simulink model "simulinkDroneDynamics"  (R2022b)
settings: Solver=VariableStepAuto  StartTime=0.0  StopTime=10.0  FixedStep=dt  RelTol=1e-3
values from neighbouring files (symbols this model uses):
  b = 0.71    [Data.m]
  g_vect = [0; 0; m*g]    [Data.m]
  Kd_vx = 0.5    [Data.m]
  Kd_vy = 0.5    [Data.m]
  Kd_vz = 1    [Data.m]
  Ki_vx = 0.5    [Data.m]
  Ki_vy = 0.5    [Data.m]
  Ki_vz = 10    [Data.m]
  Kp_vx = 5    [Data.m]
  Kp_vy = 5    [Data.m]
  Kp_vz = 15    [Data.m]
  Kp_x = 0.1    [Data.m]
  Kp_y = 0.1    [Data.m]
  Kp_z = 1    [Data.m]
  m = 3.074    [Data.m]
  mixer = [        -1         -1        -1         -1 ... (first row only)    [Data.m]
  mixer_inv = inv(mixer)    [Data.m]
  NED2ECI = [ 1  0  0 ... (first row only)    [Data.m]
  omega0 = zeros(3,1)    [Data.m]
  p0 = zeros(3,1)    [Data.m]
  q0 = [1 0 0 0]'    [Data.m]
  tau = 1/900    (= 0.00111111111111)    [Data.m]
  v0 = zeros(3,1)    [Data.m]
undefined symbols (not defined in the file or in its folder): guidance
libraries: slpidlib x3, sharedtransform x1, simulink_extras x1, sim3dlib x1, uavsim3dlib x1
settings Model: Creator=Pietro Bruschi  LastModifiedBy=Utente
settings SFSimCC: SimCustomHeaderCode="#include \"controller_vel.h\""  SimUserSources=controller_vel.c  CustomCodeGlobalsAsFunctionIO=on

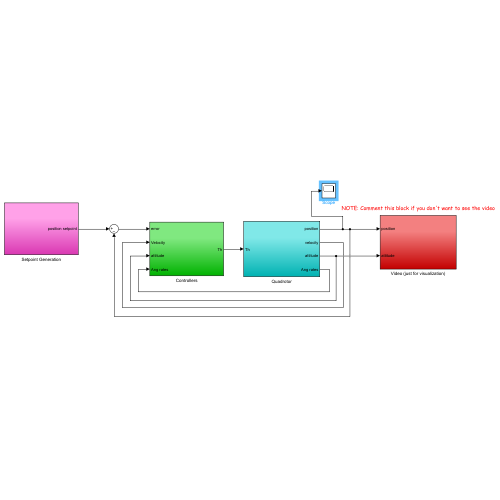
[thumbnail: Simulink's stored preview of the top-level diagram]
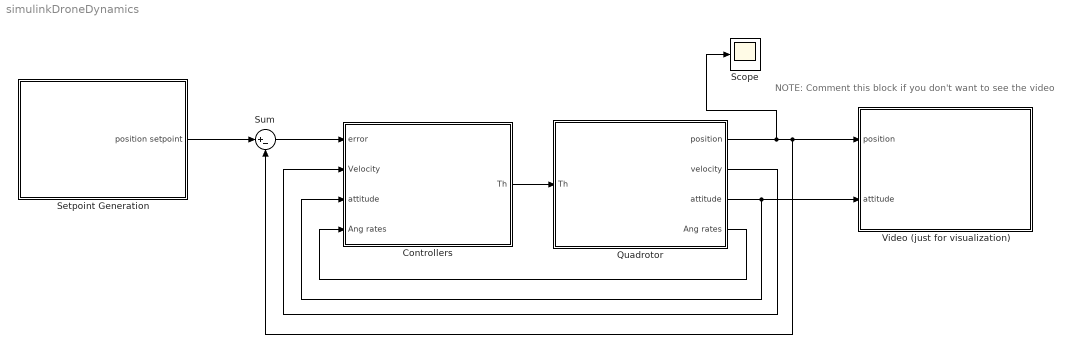
== system simulinkDroneDynamics ==
  note: NOTE: Comment this block if you don't want to see the video
  Controllers : Subsystem
  Quadrotor : Subsystem
  Scope : Scope
  Setpoint Generation : Subsystem
  Sum : Sum  Inputs=|+-
  Video (just for visualization) : Subsystem
  wires:
  Sum/1 -> Controllers/1("error ")
  Controllers/1(Th) -> Quadrotor/1(Th)
  Quadrotor/1(position) -> Scope/1, Sum/2, Video (just for visualization)/1(position)
  Setpoint Generation/1(position setpoint) -> Sum/1
  Quadrotor/4(Ang rates) -> Controllers/4(Ang rates)
  Quadrotor/3(attitude) -> Controllers/3(attitude), Video (just for visualization)/2(attitude)
  Quadrotor/2(velocity) -> Controllers/2(Velocity)

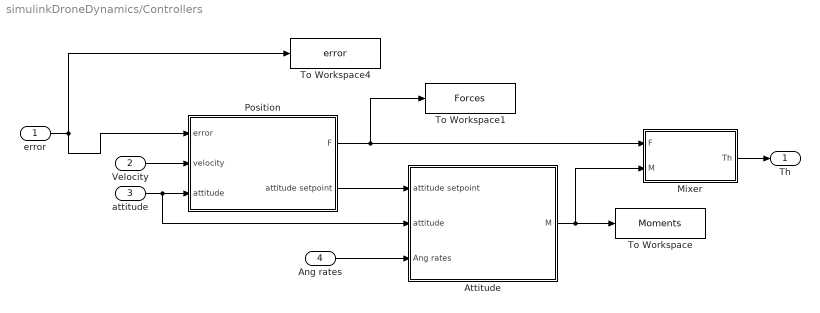
== system simulinkDroneDynamics/Controllers ==
  "error " : Inport
  Velocity : Inport  Port=2
  attitude : Inport  Port=3
  Ang rates : Inport  Port=4
  Attitude : Subsystem
  Mixer : Subsystem
  Position : Subsystem
  To Workspace : ToWorkspace  VariableName=Moments  SaveFormat=Timeseries  SampleTime=-1
  To Workspace1 : ToWorkspace  VariableName=Forces  SaveFormat=Timeseries  SampleTime=-1
  To Workspace4 : ToWorkspace  VariableName=error  SaveFormat=Timeseries  SampleTime=-1
  Th : Outport
  wires:
  Position/2(attitude setpoint) -> Attitude/1(attitude setpoint)
  Velocity/1 -> Position/2(velocity)
  Attitude/1(M) -> Mixer/2(M), To Workspace/1
  attitude/1 -> Position/3(attitude), Attitude/2(attitude)
  Ang rates/1 -> Attitude/3(Ang rates)
  Position/1(F) -> Mixer/1(F), To Workspace1/1
  Mixer/1(Th) -> Th/1
  "error "/1 -> Position/1("error "), To Workspace4/1

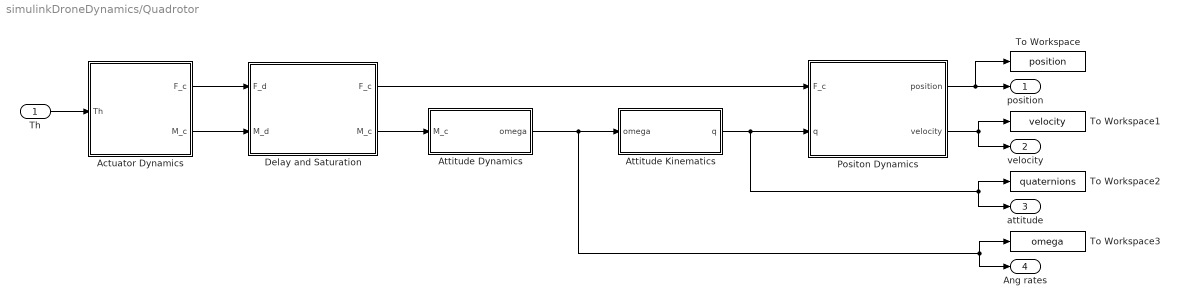
== system simulinkDroneDynamics/Quadrotor ==
  Th : Inport
  Actuator Dynamics : Subsystem
  Attitude Dynamics : Subsystem
  Attitude Kinematics : Subsystem
  Delay and Saturation : Subsystem
  Positon Dynamics : Subsystem
  To Workspace : ToWorkspace  VariableName=position  SaveFormat=Timeseries  SampleTime=-1
  To Workspace1 : ToWorkspace  VariableName=velocity  SaveFormat=Timeseries  SampleTime=-1
  To Workspace2 : ToWorkspace  VariableName=quaternions  SaveFormat=Timeseries  SampleTime=-1
  To Workspace3 : ToWorkspace  VariableName=omega  SaveFormat=Timeseries  SampleTime=-1
  position : Outport
  velocity : Outport  Port=2
  attitude : Outport  Port=3
  Ang rates : Outport  Port=4
  wires:
  Attitude Dynamics/1(omega) -> To Workspace3/1, Ang rates/1, Attitude Kinematics/1(omega)
  Attitude Kinematics/1(q) -> To Workspace2/1, attitude/1, Positon Dynamics/2(q)
  Positon Dynamics/1(position) -> To Workspace/1, position/1
  Positon Dynamics/2(velocity) -> velocity/1, To Workspace1/1
  Th/1 -> Actuator Dynamics/1(Th)
  Delay and Saturation/2(M_c) -> Attitude Dynamics/1(M_c)
  Actuator Dynamics/2(M_c) -> Delay and Saturation/2(M_d)
  Actuator Dynamics/1(F_c) -> Delay and Saturation/1(F_d)
  Delay and Saturation/1(F_c) -> Positon Dynamics/1(F_c)

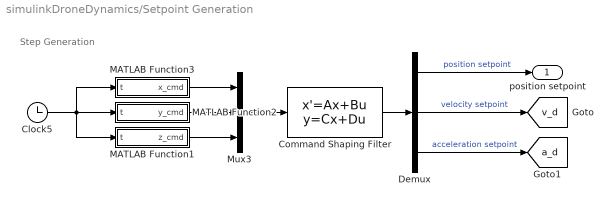
== system simulinkDroneDynamics/Setpoint Generation ==
  note: Step Generation
  Clock5 : Clock
  "Command Shaping Filter " : StateSpace  A=guidance.A_d  B=guidance.B_d  C=eye(9)  D=zeros(9,3)  InitialCondition=zeros(9,1)
  Demux : Demux  Outputs=3
  MATLAB Function1 : MATLAB Function  TreatAsAtomicUnit=on
  MATLAB Function2 : MATLAB Function  TreatAsAtomicUnit=on
  MATLAB Function3 : MATLAB Function  TreatAsAtomicUnit=on
  Mux3 : Mux  Inputs=3
  position setpoint : Outport
  tag scope: a_d=global, v_d=global
  wires:
  MATLAB Function1/1(z_cmd) -> Mux3/3
  MATLAB Function3/1(x_cmd) -> Mux3/1
  "Command Shaping Filter "/1 -> Demux/1
  Mux3/1 -> "Command Shaping Filter "/1
  MATLAB Function2/1(y_cmd) -> Mux3/2
  Clock5/1 -> MATLAB Function1/1(t), MATLAB Function2/1(t), MATLAB Function3/1(t)
  Demux/2 -> [v_d]  "velocity setpoint"
  Demux/3 -> [a_d]  "acceleration setpoint"
  Demux/1 -> position setpoint/1  "position setpoint"

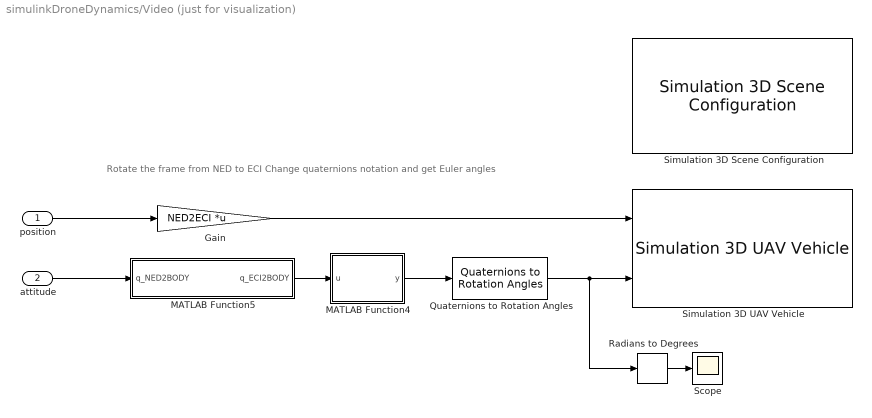
== system simulinkDroneDynamics/Video (just for visualization) ==
  note: Rotate the frame from NED to ECI
      | Change quaternions notation and get Euler angles
  position : Inport
  attitude : Inport  Port=2
  Gain : Gain  Gain=NED2ECI  Multiplication=Matrix(K*u)
  MATLAB Function4 : MATLAB Function  TreatAsAtomicUnit=on
  MATLAB Function5 : MATLAB Function  TreatAsAtomicUnit=on
  Quaternions to Rotation Angles : sharedtransform/Quaternions to Rotation Angles  rotationOrder=ZYX  aMode=aMode
  Radians to Degrees : simulink_extras/Transformations/Radians to Degrees
  Scope : Scope
  Simulation 3D Scene Configuration : sim3dlib/Simulation 3D Scene Configuration  Priority=0  ProjectFormat=Default Scenes  SceneDesc=US city block  ProjectName=C:\Program Files\MATLAB\R2022b\toolbox\shared\sim3d_projects\automotive_project\UE4\WindowsNoEditor\VehicleSimulation.exe  ScenePath=/Game/Maps/USCityBlock  EnableOpenDRIVE=off  vehTagList={'Scene Origin';'SimulinkVehicle1'}  vehTag=Scene Origin  OpVisEn=off  Ts=0.01  EnableWindow=on  EnableRemoteAccess=off  EnableWeather=off  SunAltitude=40.0  SunAzimuth=90  clouds=10  wind=1  fog=0  rain=0  EnableGeospatial=off  OriginHeight=200  OriginLatitude=40.744652  OriginLongitude=-73.988864  MapStyle=Aerial  AdditionalAssetIDs=[]  UseAdvancedSunSky=off  SolarTime=11  TimeZone=-5  Day=21  Month=9  Year=2022  UseDaylightSavingTime=on  DSTStartDay=10  DSTStartMonth=3  DSTEndDay=3  DSTEndMonth=11  DSTSwitchHour=2  sensorTag=MainCamera1  sensorId=1  sensorName=MainCamera1  mountLoc=Origin  offsetFlag=off  tmountOffset=[0, 0, 0]  rmountOffset=[0, 0, 0]  HorizontalResolution=1280  VerticalResolution=720  HorizontalFOV=60  mountPoint=[0 0 0]  mountOrientation=[0 0 0]  aMode=4  ID=1  GeoTrigger=Inactive
      settings: LibrarySourceBlock=uavsim3dlib/Simulation 3D Scene Configuration
  Simulation 3D UAV Vehicle : uavsim3dlib/Simulation 3D UAV Vehicle  Priority=-1  Mesh=Quadrotor  MeshPath=/MathWorksUAVContent/UAVs/HexaRotorUAV/HexaRotor.HexaRotor  Color=Black  ActorName=SimulinkVehicle1  InitialTranslation=[0 0 .2]  InitialRotation=[0 0 0]  SampleTime=-1  ActorType=SimulinkVehicle  ID=1  aMode=4  ActorTag=SimulinkVehicle1
  wires:
  Radians to Degrees/1 -> Scope/1
  MATLAB Function5/1(q_ECI2BODY) -> MATLAB Function4/1(u)
  position/1 -> Gain/1
  MATLAB Function4/1(y) -> Quaternions to Rotation Angles/1
  Gain/1 -> Simulation 3D UAV Vehicle/1
  attitude/1 -> MATLAB Function5/1(q_NED2BODY)
  Quaternions to Rotation Angles/1 -> Simulation 3D UAV Vehicle/2, Radians to Degrees/1

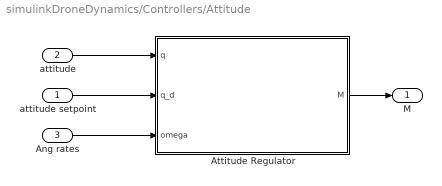
== system simulinkDroneDynamics/Controllers/Attitude ==
  attitude setpoint : Inport
  attitude : Inport  Port=2
  Ang rates : Inport  Port=3
  Attitude Regulator : MATLAB Function  TreatAsAtomicUnit=on
  M : Outport
  wires:
  attitude/1 -> Attitude Regulator/1(q)
  Attitude Regulator/1(M) -> M/1
  Ang rates/1 -> Attitude Regulator/3(omega)
  attitude setpoint/1 -> Attitude Regulator/2(q_d)

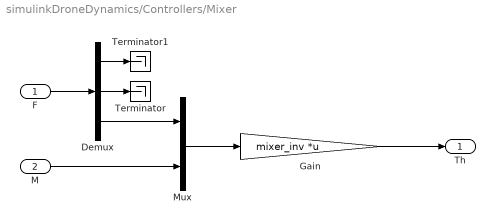
== system simulinkDroneDynamics/Controllers/Mixer ==
  F : Inport
  M : Inport  Port=2
  Demux : Demux  Outputs=3
  Gain : Gain  Gain=mixer_inv  Multiplication=Matrix(K*u) (u vector)
  Mux : Mux  Inputs=2
  Terminator : Terminator
  Terminator1 : Terminator
  Th : Outport
  wires:
  M/1 -> Mux/2
  Mux/1 -> Gain/1
  Demux/3 -> Mux/1
  F/1 -> Demux/1
  Demux/2 -> Terminator/1
  Demux/1 -> Terminator1/1
  Gain/1 -> Th/1

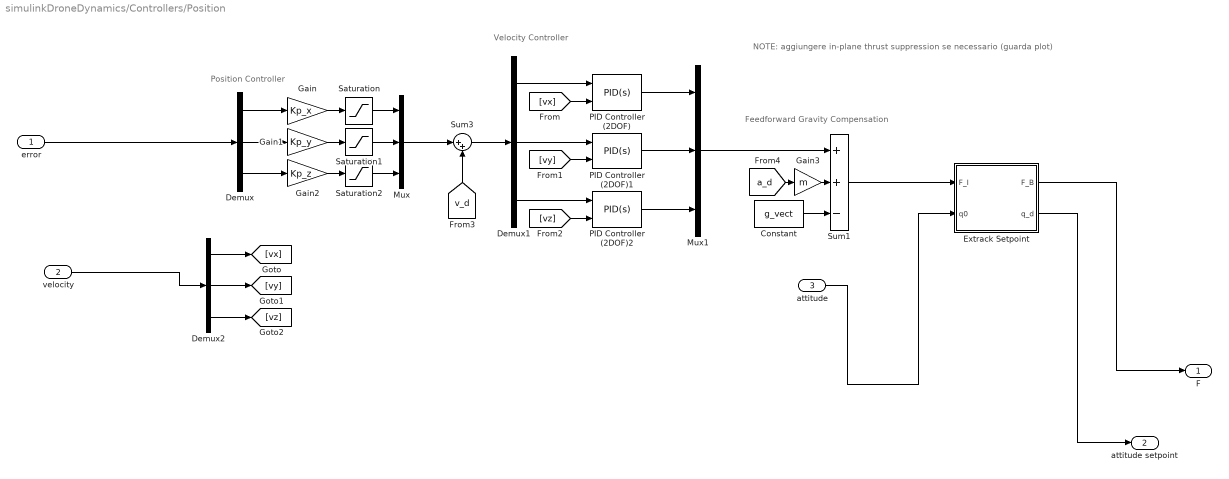
== system simulinkDroneDynamics/Controllers/Position ==
  note: Feedforward Gravity
      | Compensation
  note: NOTE: aggiungere in-plane thrust suppression se necessario (guarda plot)
  note: Velocity Controller
  note: Position Controller
  "error " : Inport
  velocity : Inport  Port=2
  attitude : Inport  Port=3
  Constant : Constant  Value=g_vect
  Demux : Demux  Outputs=3
  Demux1 : Demux  Outputs=3
  Demux2 : Demux  Outputs=3
  Extrack Setpoint : MATLAB Function  TreatAsAtomicUnit=on
  Gain : Gain  Gain=Kp_x
  Gain1 : Gain  Gain=Kp_y
  Gain2 : Gain  Gain=Kp_z
  Gain3 : Gain  Gain=m
  Mux : Mux  Inputs=3
  Mux1 : Mux  Inputs=3
  PID Controller (2DOF) : slpidlib/PID Controller (2DOF)  Controller=PID  Form=Parallel  TimeDomain=Continuous-time  UseExternalTs=off  SampleTime=-1  IntegratorMethod=Forward Euler  FilterMethod=Forward Euler  ControllerParametersSource=internal  P=Kp_vx  I=Ki_vx  UseKiTs=off  D=Kd_vx  N=100  UseFilter=on  b=1  c=0  TunerSelectOption=Frequency Response Based  InitialConditionSource=internal  InitialConditionForIntegrator=0  InitialConditionForFilter=0  DifferentiatorICPrevScaledInput=0  ExternalReset=none  TrackingMode=off  Kt=1  LimitOutput=off  SatLimitsSource=internal  UpperSaturationLimit=inf  LowerSaturationLimit=-inf  LinearizeAsGain=on  AntiWindupMode=none  Kb=1  LimitIntegrator=off  UpperIntegratorSaturationLimit=inf  LowerIntegratorSaturationLimit=-inf  POutMin=[]  POutMax=[]  IOutMin=[]  IOutMax=[]  DOutMin=[]  DOutMax=[]  NOutMin=[]  NOutMax=[]  bOutMin=[]  bOutMax=[]  cOutMin=[]  cOutMax=[]  SumOutMin=[]  SumOutMax=[]  SaturationOutMin=[]  SaturationOutMax=[]  PParamMin=[]  PParamMax=[]  IParamMin=[]  IParamMax=[]  DParamMin=[]  DParamMax=[]  NParamMin=[]  NParamMax=[]  bParamMin=[]  bParamMax=[]  cParamMin=[]  cParamMax=[]  KbParamMin=[]  KbParamMax=[]  KtParamMin=[]  KtParamMax=[]  KbOutMin=[]  KbOutMax=[]  KtOutMin=[]  KtOutMax=[]  IntegratorOutMin=[]  IntegratorOutMax=[]  FilterOutMin=[]  FilterOutMax=[]  SumI1OutMin=[]  SumI1OutMax=[]  SumI2OutMin=[]  SumI2OutMax=[]  SumI3OutMin=[]  SumI3OutMax=[]  SumI4OutMin=[]  SumI4OutMax=[]  SumDOutMin=[]  SumDOutMax=[]  Sum1OutMin=[]  Sum1OutMax=[]  Sum2OutMin=[]  Sum2OutMax=[]  Sum3OutMin=[]  Sum3OutMax=[]  DifferentiatorOutMin=[]  DifferentiatorOutMax=[]  FilterDiffOutCoefMin=[]  FilterDiffOutCoefMax=[]  ReciprocalOutMin=[]  ReciprocalOutMax=[]  SumDenOutMin=[]  SumDenOutMax=[]  SumNumOutMin=[]  SumNumOutMax=[]  DivideOutMin=[]  DivideOutMax=[]  UdiffTsProdOutMin=[]  UdiffTsProdOutMax=[]  NTsProdOutMin=[]  NTsProdOutMax=[]  UintegralTsProdOutMin=[]  UintegralTsProdOutMax=[]  UngainTsProdOutMin=[]  UngainTsProdOutMax=[]  ClampingZeroOutDataTypeStr=Inherit: Inherit via back propagation  ClampingZeroOutMin=[]  ClampingZeroOutMax=[]  FilterDenConstantOutDataTypeStr=Inherit: Inherit via back propagation  FilterDenConstantOutMin=[]  FilterDenConstantOutMax=[]  PCopyOutDataTypeStr=Inherit: Inherit via back propagation  PCopyOutMin=[]  PCopyOutMax=[]  NCopyOutDataTypeStr=Inherit: Inherit via back propagation  NCopyOutMin=[]  NCopyOutMax=[]  IntegratorContinuousStateAttributes=''  IntegratorStateMustResolveToSignalObject=off  IntegratorRTWStateStorageClass=Auto  FilterContinuousStateAttributes=''  FilterStateMustResolveToSignalObject=off  FilterRTWStateStorageClass=Auto  ParallelPVariant=InternalParameters  IdealPVariant=Disabled  IVariant=InternalParameters  DVariant=InternalParameters  bVariant=InternalParameters  cVariant=InternalParameters  IntegratorVariant=Continuous  SatVariant=Disabled  AWVariant=Passthrough  PCopyVariant=Disabled  TRVariant=Disabled  FdbkBlocksVariant=Forward  IdealPFdbkVariant=Disabled  SatFdbkVariant=Disabled  DerivativeFilterVariant=ContFilter  NVariant=InternalParameters  NCopyVariant=Disabled  FilterICVariant=InternalICsFilter  IntegratorICVariant=InternalICs  ExternalResetVariant=Disabled  TRSumVariant=Passthrough  SumFdbkVariant=Disabled  SumVariant=Sum_PID  TsampFilterVariant=InternalTs  TsampNgainVariant=Passthrough  TsampIntegralVariant=Passthrough  ExternalSaturationOutDataTypeStr=Inherit: Same as second input
  PID Controller (2DOF)1 : slpidlib/PID Controller (2DOF)  Controller=PID  Form=Parallel  TimeDomain=Continuous-time  UseExternalTs=off  SampleTime=-1  IntegratorMethod=Forward Euler  FilterMethod=Forward Euler  ControllerParametersSource=internal  P=Kp_vy  I=Ki_vy  UseKiTs=off  D=Kd_vy  N=100  UseFilter=on  b=1  c=0  TunerSelectOption=Frequency Response Based  InitialConditionSource=internal  InitialConditionForIntegrator=0  InitialConditionForFilter=0  DifferentiatorICPrevScaledInput=0  ExternalReset=none  TrackingMode=off  Kt=1  LimitOutput=off  SatLimitsSource=internal  UpperSaturationLimit=inf  LowerSaturationLimit=-inf  LinearizeAsGain=on  AntiWindupMode=none  Kb=1  LimitIntegrator=off  UpperIntegratorSaturationLimit=inf  LowerIntegratorSaturationLimit=-inf  POutMin=[]  POutMax=[]  IOutMin=[]  IOutMax=[]  DOutMin=[]  DOutMax=[]  NOutMin=[]  NOutMax=[]  bOutMin=[]  bOutMax=[]  cOutMin=[]  cOutMax=[]  SumOutMin=[]  SumOutMax=[]  SaturationOutMin=[]  SaturationOutMax=[]  PParamMin=[]  PParamMax=[]  IParamMin=[]  IParamMax=[]  DParamMin=[]  DParamMax=[]  NParamMin=[]  NParamMax=[]  bParamMin=[]  bParamMax=[]  cParamMin=[]  cParamMax=[]  KbParamMin=[]  KbParamMax=[]  KtParamMin=[]  KtParamMax=[]  KbOutMin=[]  KbOutMax=[]  KtOutMin=[]  KtOutMax=[]  IntegratorOutMin=[]  IntegratorOutMax=[]  FilterOutMin=[]  FilterOutMax=[]  SumI1OutMin=[]  SumI1OutMax=[]  SumI2OutMin=[]  SumI2OutMax=[]  SumI3OutMin=[]  SumI3OutMax=[]  SumI4OutMin=[]  SumI4OutMax=[]  SumDOutMin=[]  SumDOutMax=[]  Sum1OutMin=[]  Sum1OutMax=[]  Sum2OutMin=[]  Sum2OutMax=[]  Sum3OutMin=[]  Sum3OutMax=[]  DifferentiatorOutMin=[]  DifferentiatorOutMax=[]  FilterDiffOutCoefMin=[]  FilterDiffOutCoefMax=[]  ReciprocalOutMin=[]  ReciprocalOutMax=[]  SumDenOutMin=[]  SumDenOutMax=[]  SumNumOutMin=[]  SumNumOutMax=[]  DivideOutMin=[]  DivideOutMax=[]  UdiffTsProdOutMin=[]  UdiffTsProdOutMax=[]  NTsProdOutMin=[]  NTsProdOutMax=[]  UintegralTsProdOutMin=[]  UintegralTsProdOutMax=[]  UngainTsProdOutMin=[]  UngainTsProdOutMax=[]  ClampingZeroOutDataTypeStr=Inherit: Inherit via back propagation  ClampingZeroOutMin=[]  ClampingZeroOutMax=[]  FilterDenConstantOutDataTypeStr=Inherit: Inherit via back propagation  FilterDenConstantOutMin=[]  FilterDenConstantOutMax=[]  PCopyOutDataTypeStr=Inherit: Inherit via back propagation  PCopyOutMin=[]  PCopyOutMax=[]  NCopyOutDataTypeStr=Inherit: Inherit via back propagation  NCopyOutMin=[]  NCopyOutMax=[]  IntegratorContinuousStateAttributes=''  IntegratorStateMustResolveToSignalObject=off  IntegratorRTWStateStorageClass=Auto  FilterContinuousStateAttributes=''  FilterStateMustResolveToSignalObject=off  FilterRTWStateStorageClass=Auto  ParallelPVariant=InternalParameters  IdealPVariant=Disabled  IVariant=InternalParameters  DVariant=InternalParameters  bVariant=InternalParameters  cVariant=InternalParameters  IntegratorVariant=Continuous  SatVariant=Disabled  AWVariant=Passthrough  PCopyVariant=Disabled  TRVariant=Disabled  FdbkBlocksVariant=Forward  IdealPFdbkVariant=Disabled  SatFdbkVariant=Disabled  DerivativeFilterVariant=ContFilter  NVariant=InternalParameters  NCopyVariant=Disabled  FilterICVariant=InternalICsFilter  IntegratorICVariant=InternalICs  ExternalResetVariant=Disabled  TRSumVariant=Passthrough  SumFdbkVariant=Disabled  SumVariant=Sum_PID  TsampFilterVariant=InternalTs  TsampNgainVariant=Passthrough  TsampIntegralVariant=Passthrough  ExternalSaturationOutDataTypeStr=Inherit: Same as second input
  PID Controller (2DOF)2 : slpidlib/PID Controller (2DOF)  Controller=PID  Form=Parallel  TimeDomain=Continuous-time  UseExternalTs=off  SampleTime=-1  IntegratorMethod=Forward Euler  FilterMethod=Forward Euler  ControllerParametersSource=internal  P=Kp_vz  I=Ki_vz  UseKiTs=off  D=Kd_vz  N=100  UseFilter=on  b=1  c=0  TunerSelectOption=Frequency Response Based  InitialConditionSource=internal  InitialConditionForIntegrator=0  InitialConditionForFilter=0  DifferentiatorICPrevScaledInput=0  ExternalReset=none  TrackingMode=off  Kt=1  LimitOutput=off  SatLimitsSource=internal  UpperSaturationLimit=inf  LowerSaturationLimit=-inf  LinearizeAsGain=on  AntiWindupMode=none  Kb=1  LimitIntegrator=off  UpperIntegratorSaturationLimit=inf  LowerIntegratorSaturationLimit=-inf  POutMin=[]  POutMax=[]  IOutMin=[]  IOutMax=[]  DOutMin=[]  DOutMax=[]  NOutMin=[]  NOutMax=[]  bOutMin=[]  bOutMax=[]  cOutMin=[]  cOutMax=[]  SumOutMin=[]  SumOutMax=[]  SaturationOutMin=[]  SaturationOutMax=[]  PParamMin=[]  PParamMax=[]  IParamMin=[]  IParamMax=[]  DParamMin=[]  DParamMax=[]  NParamMin=[]  NParamMax=[]  bParamMin=[]  bParamMax=[]  cParamMin=[]  cParamMax=[]  KbParamMin=[]  KbParamMax=[]  KtParamMin=[]  KtParamMax=[]  KbOutMin=[]  KbOutMax=[]  KtOutMin=[]  KtOutMax=[]  IntegratorOutMin=[]  IntegratorOutMax=[]  FilterOutMin=[]  FilterOutMax=[]  SumI1OutMin=[]  SumI1OutMax=[]  SumI2OutMin=[]  SumI2OutMax=[]  SumI3OutMin=[]  SumI3OutMax=[]  SumI4OutMin=[]  SumI4OutMax=[]  SumDOutMin=[]  SumDOutMax=[]  Sum1OutMin=[]  Sum1OutMax=[]  Sum2OutMin=[]  Sum2OutMax=[]  Sum3OutMin=[]  Sum3OutMax=[]  DifferentiatorOutMin=[]  DifferentiatorOutMax=[]  FilterDiffOutCoefMin=[]  FilterDiffOutCoefMax=[]  ReciprocalOutMin=[]  ReciprocalOutMax=[]  SumDenOutMin=[]  SumDenOutMax=[]  SumNumOutMin=[]  SumNumOutMax=[]  DivideOutMin=[]  DivideOutMax=[]  UdiffTsProdOutMin=[]  UdiffTsProdOutMax=[]  NTsProdOutMin=[]  NTsProdOutMax=[]  UintegralTsProdOutMin=[]  UintegralTsProdOutMax=[]  UngainTsProdOutMin=[]  UngainTsProdOutMax=[]  ClampingZeroOutDataTypeStr=Inherit: Inherit via back propagation  ClampingZeroOutMin=[]  ClampingZeroOutMax=[]  FilterDenConstantOutDataTypeStr=Inherit: Inherit via back propagation  FilterDenConstantOutMin=[]  FilterDenConstantOutMax=[]  PCopyOutDataTypeStr=Inherit: Inherit via back propagation  PCopyOutMin=[]  PCopyOutMax=[]  NCopyOutDataTypeStr=Inherit: Inherit via back propagation  NCopyOutMin=[]  NCopyOutMax=[]  IntegratorContinuousStateAttributes=''  IntegratorStateMustResolveToSignalObject=off  IntegratorRTWStateStorageClass=Auto  FilterContinuousStateAttributes=''  FilterStateMustResolveToSignalObject=off  FilterRTWStateStorageClass=Auto  ParallelPVariant=InternalParameters  IdealPVariant=Disabled  IVariant=InternalParameters  DVariant=InternalParameters  bVariant=InternalParameters  cVariant=InternalParameters  IntegratorVariant=Continuous  SatVariant=Disabled  AWVariant=Passthrough  PCopyVariant=Disabled  TRVariant=Disabled  FdbkBlocksVariant=Forward  IdealPFdbkVariant=Disabled  SatFdbkVariant=Disabled  DerivativeFilterVariant=ContFilter  NVariant=InternalParameters  NCopyVariant=Disabled  FilterICVariant=InternalICsFilter  IntegratorICVariant=InternalICs  ExternalResetVariant=Disabled  TRSumVariant=Passthrough  SumFdbkVariant=Disabled  SumVariant=Sum_PID  TsampFilterVariant=InternalTs  TsampNgainVariant=Passthrough  TsampIntegralVariant=Passthrough  ExternalSaturationOutDataTypeStr=Inherit: Same as second input
  Saturation : Saturate  UpperLimit=10  LowerLimit=-10
  Saturation1 : Saturate  UpperLimit=10  LowerLimit=-10
  Saturation2 : Saturate  UpperLimit=10  LowerLimit=-10
  Sum1 : Sum  Inputs=++-
  Sum3 : Sum  Inputs=|++
  F : Outport
  attitude setpoint : Outport  Port=2
  wires:
  Demux/1 -> Gain/1
  Demux/2 -> Gain1/1
  Demux/3 -> Gain2/1
  Demux2/1 -> [vx]
  Demux2/2 -> [vy]
  Demux2/3 -> [vz]
  "error "/1 -> Demux/1
  velocity/1 -> Demux2/1
  attitude/1 -> Extrack Setpoint/2(q0)
  Gain1/1 -> Saturation1/1
  Gain2/1 -> Saturation2/1
  Gain/1 -> Saturation/1
  Sum1/1 -> Extrack Setpoint/1(F_I)
  PID Controller (2DOF)1/1 -> Mux1/2
  Demux1/2 -> PID Controller (2DOF)1/1
  [vy] -> PID Controller (2DOF)1/2
  Saturation1/1 -> Mux/2
  Saturation2/1 -> Mux/3
  Saturation/1 -> Mux/1
  Mux/1 -> Sum3/1
  Sum3/1 -> Demux1/1
  [v_d] -> Sum3/2
  Constant/1 -> Sum1/3
  Gain3/1 -> Sum1/2
  [a_d] -> Gain3/1
  PID Controller (2DOF)2/1 -> Mux1/3
  Demux1/3 -> PID Controller (2DOF)2/1
  [vz] -> PID Controller (2DOF)2/2
  Mux1/1 -> Sum1/1
  PID Controller (2DOF)/1 -> Mux1/1
  Demux1/1 -> PID Controller (2DOF)/1
  [vx] -> PID Controller (2DOF)/2
  Extrack Setpoint/1(F_B) -> F/1
  Extrack Setpoint/2(q_d) -> attitude setpoint/1

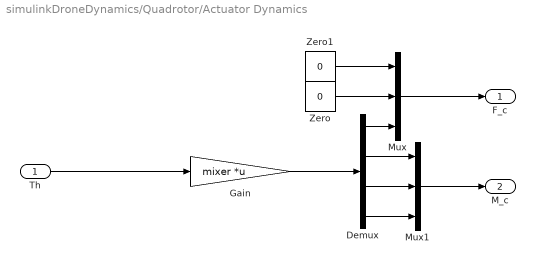
== system simulinkDroneDynamics/Quadrotor/Actuator Dynamics ==
  Th : Inport
  Demux : Demux
  Gain : Gain  Gain=mixer  Multiplication=Matrix(K*u) (u vector)
  Mux : Mux  Inputs=3
  Mux1 : Mux  Inputs=3
  Zero : Constant  Value=0  OutDataTypeStr=Inherit: Inherit via back propagation
  Zero1 : Constant  Value=0  OutDataTypeStr=Inherit: Inherit via back propagation
  F_c : Outport
  M_c : Outport  Port=2
  wires:
  Gain/1 -> Demux/1
  Mux/1 -> F_c/1
  Demux/1 -> Mux/3
  Zero1/1 -> Mux/1
  Zero/1 -> Mux/2
  Mux1/1 -> M_c/1
  Demux/2 -> Mux1/1
  Demux/3 -> Mux1/2
  Demux/4 -> Mux1/3
  Th/1 -> Gain/1

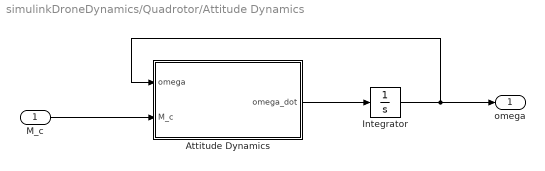
== system simulinkDroneDynamics/Quadrotor/Attitude Dynamics ==
  M_c : Inport
  Attitude Dynamics : MATLAB Function  TreatAsAtomicUnit=on
  Integrator : Integrator  InitialCondition=omega0
  omega : Outport
  wires:
  M_c/1 -> Attitude Dynamics/2(M_c)
  Attitude Dynamics/1(omega_dot) -> Integrator/1
  Integrator/1 -> Attitude Dynamics/1(omega), omega/1

== system simulinkDroneDynamics/Quadrotor/Attitude Kinematics ==
  omega : Inport
  Integrator : Integrator  InitialCondition=q0
  MATLAB Function : MATLAB Function  TreatAsAtomicUnit=on
  q : Outport
  wires:
  Integrator/1 -> MATLAB Function/1(q), q/1
  omega/1 -> MATLAB Function/2(omega)
  MATLAB Function/1(q_dot) -> Integrator/1

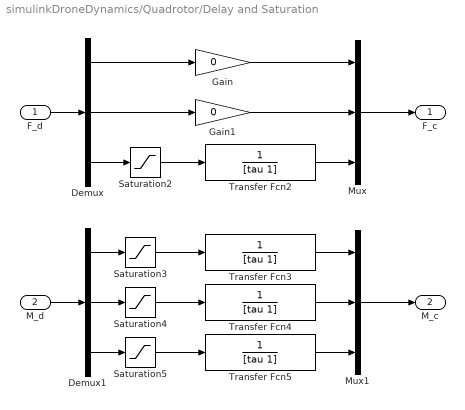
== system simulinkDroneDynamics/Quadrotor/Delay and Saturation ==
  F_d : Inport
  M_d : Inport  Port=2
  Demux : Demux  Outputs=3
  Demux1 : Demux  Outputs=3
  Gain : Gain  Gain=0
  Gain1 : Gain  Gain=0
  Mux : Mux  Inputs=3
  Mux1 : Mux  Inputs=3
  Saturation2 : Saturate  UpperLimit=250  LowerLimit=-250
  Saturation3 : Saturate  UpperLimit=250*b  LowerLimit=-250*b
  Saturation4 : Saturate  UpperLimit=250*b  LowerLimit=-250*b
  Saturation5 : Saturate  UpperLimit=250*b  LowerLimit=-250*b
  Transfer Fcn{2..5} (4 alike) : TransferFcn  Denominator=[tau 1]
  F_c : Outport
  M_c : Outport  Port=2
  wires:
  F_d/1 -> Demux/1
  Mux/1 -> F_c/1
  Gain/1 -> Mux/1
  Gain1/1 -> Mux/2
  Mux1/1 -> M_c/1
  M_d/1 -> Demux1/1
  Demux/2 -> Gain1/1
  Demux/1 -> Gain/1
  Transfer Fcn4/1 -> Mux1/2
  Transfer Fcn5/1 -> Mux1/3
  Transfer Fcn2/1 -> Mux/3
  Transfer Fcn3/1 -> Mux1/1
  Demux/3 -> Saturation2/1
  Demux1/1 -> Saturation3/1
  Demux1/2 -> Saturation4/1
  Demux1/3 -> Saturation5/1
  Saturation2/1 -> Transfer Fcn2/1
  Saturation5/1 -> Transfer Fcn5/1
  Saturation4/1 -> Transfer Fcn4/1
  Saturation3/1 -> Transfer Fcn3/1

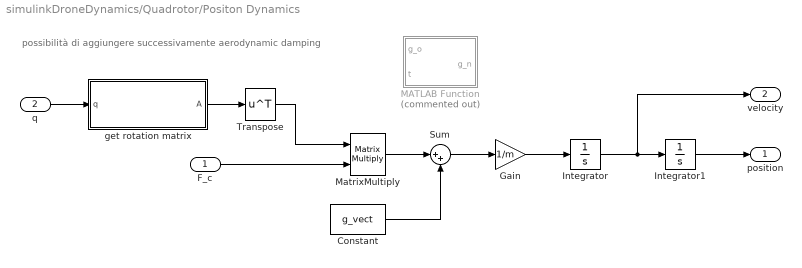
== system simulinkDroneDynamics/Quadrotor/Positon Dynamics ==
  note: possibilità di aggiungere successivamente aerodynamic damping
  F_c : Inport
  q : Inport  Port=2
  Constant : Constant  Value=g_vect
  Gain : Gain  Gain=1/m
  Integrator : Integrator  InitialCondition=v0
  Integrator1 : Integrator  InitialCondition=p0
  MATLAB Function : MATLAB Function  Commented=on  TreatAsAtomicUnit=on
  MatrixMultiply : Product  Multiplication=Matrix(*)
  Sum : Sum  Inputs=|++
  Transpose : Math  Operator=transpose
  get rotation matrix : MATLAB Function  TreatAsAtomicUnit=on
  position : Outport
  velocity : Outport  Port=2
  wires:
  Integrator/1 -> velocity/1, Integrator1/1
  Gain/1 -> Integrator/1
  MatrixMultiply/1 -> Sum/1
  q/1 -> get rotation matrix/1(q)
  get rotation matrix/1(A) -> Transpose/1
  Integrator1/1 -> position/1
  Sum/1 -> Gain/1
  F_c/1 -> MatrixMultiply/2
  Transpose/1 -> MatrixMultiply/1
  Constant/1 -> Sum/2

== matlab function simulinkDroneDynamics/Quadrotor/Attitude Kinematics/MATLAB Function ==
  data: q input; q_dot output; omega input
function q_dot = fcn(q, omega)

q = q/norm(q);

Omega = [       0   omega(3) -omega(2) omega(1) ;
         -omega(3)        0   omega(1) omega(2) ;
          omega(2) -omega(1)        0  omega(3) ;
         -omega(1) -omega(2) -omega(3)       0  ];

q_dot = 1/2 * Omega * q;

== matlab function simulinkDroneDynamics/Quadrotor/Attitude Dynamics/Attitude Dynamics ==
  data: omega input; omega_dot output; M_c input; Drone parameter
function omega_dot = fcn(omega, M_c, Drone)

J = Drone.J;
Jinv = Drone.Jinv;

omega_dot = Jinv * (-cross(omega,J*omega) + M_c);

== matlab function simulinkDroneDynamics/Quadrotor/Positon Dynamics/get rotation matrix ==
  data: q input; A output
function A = fcn(q)

q = q/norm(q);

q_v = q(1:3);

q_cross = [     0 -q(3)  q(2) ;
             q(3)     0 -q(1) ;
            -q(2)  q(1)     0 ];

A = (q(4) - q_v'*q_v)*eye(3) + 2*q_v*q_v' - 2*q(4)*q_cross;

% A = quat2dcm(q);

== matlab function simulinkDroneDynamics/Controllers/Position/Extrack Setpoint ==
  data: F_I input; F_B output; q0 input; q_d output
function [F_B, q_d] = fcn(F_I, q0)

q = q0/norm(q0);

q_v = q(1:3);

q_cross = [     0 -q(3)  q(2) ;
             q(3)     0 -q(1) ;
            -q(2)  q(1)     0 ];

A = (q(4) - q_v'*q_v)*eye(3) + 2*q_v*q_v' - 2*q(4)*q_cross;

% A = quat2dcm(q0);

b1_d = A'*[1 0 0]';
b3 = F_I / norm(F_I);
b2_c = cross(b3,b1_d);
b2 = b2_c / norm(b2_c);
b1 = cross(b2,b3);

R = [b1 b2 b3];

R = R';

vector = [R(1,1), R(2,2), R(3,3), trace(R)];
[M, i] = max(vector);

switch i
    case 1
        q_d = [ 1 + R(1,1) - R(2,2) - R(3,3);
            R(1,2) + R(2,1);
            R(1,3) + R(3,1);
            R(2,3) - R(3,2)];
        
    case 2
        q_d = [R(2,1) + R(1,2);
            1 + R(2,2) - R(3,3) - R(1,1);
            R(2,3) + R(3,2);
            R(3,1) - R(1,3)];
        
    case 3
        q_d = [R(3,1) + R(1,3);
            R(3,2) + R(2,3);
            1 + R(3,3) - R(1,1) - R(2,2);
            R(1,2) - R(2,1)];
        
    case 4
        q_d = [R(2,3) - R(3,2);
            R(3,1) - R(1,3);
            R(1,2) - R(2,1);
            1 + R(1,1) + R(2,2) + R(3,3)];
        
    otherwise
        error('Check the Attitude matrix');
end

q_d = q_d / norm(q_d);

F_B = R*F_I;

== matlab function simulinkDroneDynamics/Controllers/Attitude/Attitude Regulator ==
  data: q input; M output; q_d input; omega input; Controllers parameter
function M = fcn(q, q_d, omega, Controllers)

Kp_roll = Controllers.Kp_roll;
Kp_pitch = Controllers.Kp_pitch;
Kp_yaw = Controllers.Kp_yaw;
Kd_roll = Controllers.Kd_roll;
Kd_pitch = Controllers.Kd_pitch;
Kd_yaw = Controllers.Kd_yaw;

q_conj = [-q_d(1:3); q_d(4)];

Q = [  q(4)  q(3) -q(2)  q(1) ;
      -q(3)  q(4)  q(1)  q(2) ;
       q(2) -q(1)  q(4)  q(3) ; 
      -q(1) -q(2) -q(3)  q(4) ];

q_e = Q * q_conj;
q_e = q_e / norm(q_e);

M_x = 2*Kp_roll*(q_e(1)*q_e(4)) + Kd_roll*omega(1);
M_y = 2*Kp_pitch*(q_e(2)*q_e(4)) + Kd_pitch*omega(2);
M_z = 2*Kp_yaw*(q_e(3)*q_e(4)) + Kd_yaw*omega(3);

M = -[M_x M_y M_z]';

== matlab function simulinkDroneDynamics/Quadrotor/Positon Dynamics/MATLAB Function ==
  data: g_o input; g_n output; t input
function g_n = fcn(g_o,t)

g_n = g_o*(t>5);

== matlab function simulinkDroneDynamics/Setpoint Generation/MATLAB Function2 ==
  data: t input; y_cmd output
function y_cmd = fcn(t)

y_cmd = 0*(t<=15) - 1*(t>15);

== matlab function simulinkDroneDynamics/Setpoint Generation/MATLAB Function3 ==
  data: t input; x_cmd output
function x_cmd = fcn(t)

x_cmd = 0*(t<=10) + 1*(t>10);

== matlab function simulinkDroneDynamics/Setpoint Generation/MATLAB Function1 ==
  data: t input; z_cmd output
function z_cmd = fcn(t)

z_cmd = 0*(t<=5) - 1*(t>5);

== matlab function simulinkDroneDynamics/Video (just for visualization)/MATLAB Function4 ==
  data: u input; y output
function y = fcn(u)

% Convert from 1234 to 0123 notation

y = zeros(4,1);

y(1) = u(4);
y(2:4) = u(1:3);

== matlab function simulinkDroneDynamics/Video (just for visualization)/MATLAB Function5 ==
  data: q_NED2BODY input; q_ECI2BODY output
function q_ECI2BODY = fcn(q_NED2BODY)

% Convert quaternions from NED to ECI frames

q_ECI2NED = [ -1 0 0 0 ]';

% qv1 = [q_ECI2NED(1), q_ECI2NED(2), q_ECI2NED(3)]';
% qs1 = q_ECI2NED(4);
% 
% qv2 = [q_NED2BODY(1), q_NED2BODY(2), q_NED2BODY(3)]';
% qs2 = q_NED2BODY(4);
% 
% q_ECI2BODY = [qs1 * qv2 + qs2 * qv1 - cross( qv1, qv2 ) ;
%               qs1 * qs2 - dot( qv1, qv2 )        ];

Q = [  q_NED2BODY(4)  q_NED2BODY(3) -q_NED2BODY(2)  q_NED2BODY(1) ;
      -q_NED2BODY(3)  q_NED2BODY(4)  q_NED2BODY(1)  q_NED2BODY(2) ;
       q_NED2BODY(2) -q_NED2BODY(1)  q_NED2BODY(4)  q_NED2BODY(3) ; 
      -q_NED2BODY(1) -q_NED2BODY(2) -q_NED2BODY(3)  q_NED2BODY(4) ];

q_ECI2BODY = Q * q_ECI2NED;
q_ECI2BODY = q_ECI2BODY / norm(q_ECI2BODY);
